simulink model "Velocity_Open_loop"  (R2023a)
settings: Solver=FixedStepAuto  StartTime=0.0  StopTime=10  FixedStep=0.04  RelTol=1e-3
undefined symbols (not defined in the file): Angular, Linear
libraries: robotlib x7
settings Model: Creator=yoav  LastModifiedBy=connectlab
settings OptimizationCC: EnhancedBackFolding=on  PassReuseOutputArgsAs=Individual arguments  ZeroExternalMemoryAtStartup=off  ZeroInternalMemoryAtStartup=off  MaxStackSize=64  OptimizeBlockOrder=speed  DifferentSizesBufferReuse=on  OptimizationCustomize=off  EfficientTunableParamExpr=on
settings DebuggingCC: ParameterTunabilityLossMsg=error
settings HardwareCC: ProdBitPerPointer=32  ProdBitPerSizeT=32  ProdBitPerPtrDiffT=32  ProdLargestAtomicFloat=None  ProdIntDivRoundTo=Undefined  ProdEndianess=Unspecified  ProdWordSize=32  ProdHWDeviceType=Generic->Unspecified (assume 32-bit Generic)
settings SFSimCC: MATLABDynamicMemAlloc=off
settings RTWCC: Description=Embedded Coder  SystemTargetFile=ert.tlc  HardwareBoard=Robot Operating System (ROS)  TLCOptions="-aInlineSetEventsForThisBaseRateFcn=TLC_FALSE -aSuppressMultiTaskScheduler=TLC_FALSE  -aRateBasedStepFcn=0"  TemplateMakefile=ert_default_tmf  Toolchain=Catkin  TargetLang=C++
settings CodeAppCC: ForceParamTrailComments=on  IgnoreCustomStorageClasses=off  OperatorAnnotations=on  SimulinkDataObjDesc=on  SFDataObjDesc=on  InsertBlockDesc=on
settings ERTTargetCC: ExtMode=on  ExtModeMexArgs='192.168.1.155' 0 17725

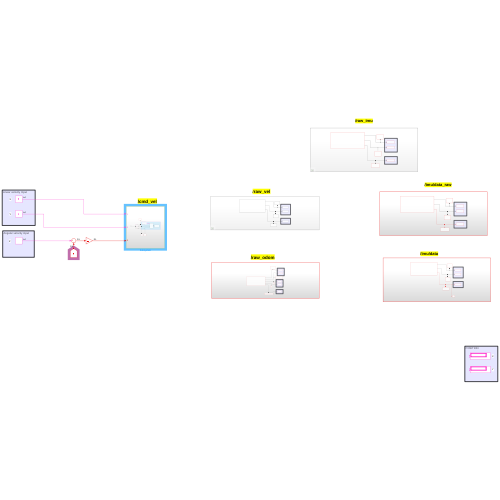
[thumbnail: Simulink's stored preview of the top-level diagram]
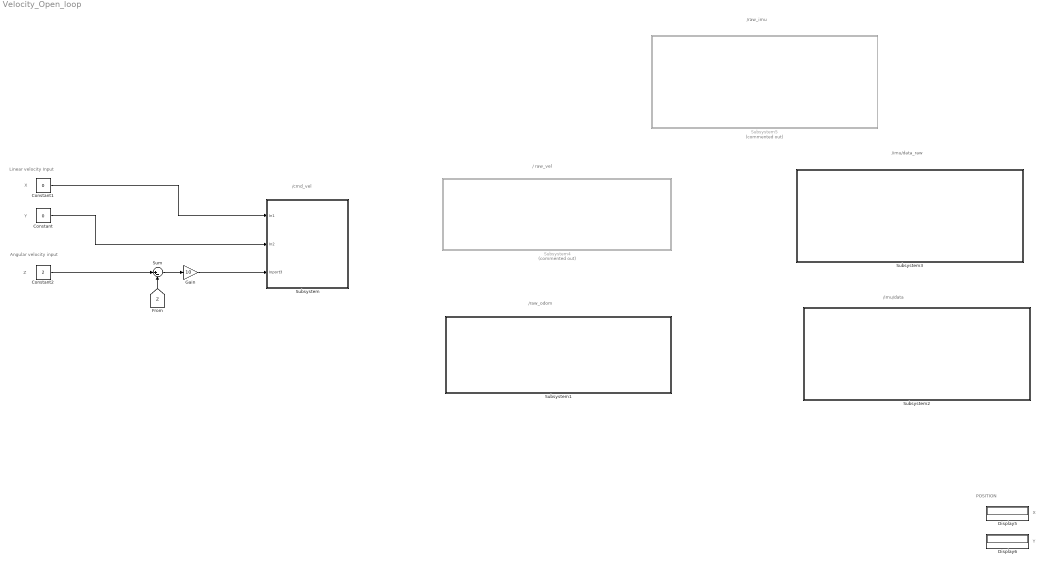
== system Velocity_Open_loop ==
  note: /raw_odom
  note: / raw_vel
  note: X
  note: Y
  note: Z
  note: Linear velocity Input
  note: Angular velocity input
  note: X
  note: POSITION
  note: Y
  note: /cmd_vel
  note: /imu/data_raw
  note: /imu/data
  note: /raw_imu
  Constant : Constant  Value=0
  Constant1 : Constant  Value=0
  Constant2 : Constant  Value=2
  Display5 : Display
  Display6 : Display
  Gain : Gain  Gain=10
  Subsystem : Subsystem
  Subsystem1 : Subsystem
  Subsystem2 : Subsystem
  Subsystem3 : Subsystem
  Subsystem4 : Subsystem  Commented=on
  Subsystem5 : Subsystem  Commented=on
  Sum : Sum  Inputs=|+-
  wires:
  Constant1/1 -> Subsystem/1(In1)
  Constant/1 -> Subsystem/2(In2)
  [Z] -> Sum/2
  Constant2/1 -> Sum/1
  Sum/1 -> Gain/1
  Gain/1 -> Subsystem/3(Inport3)

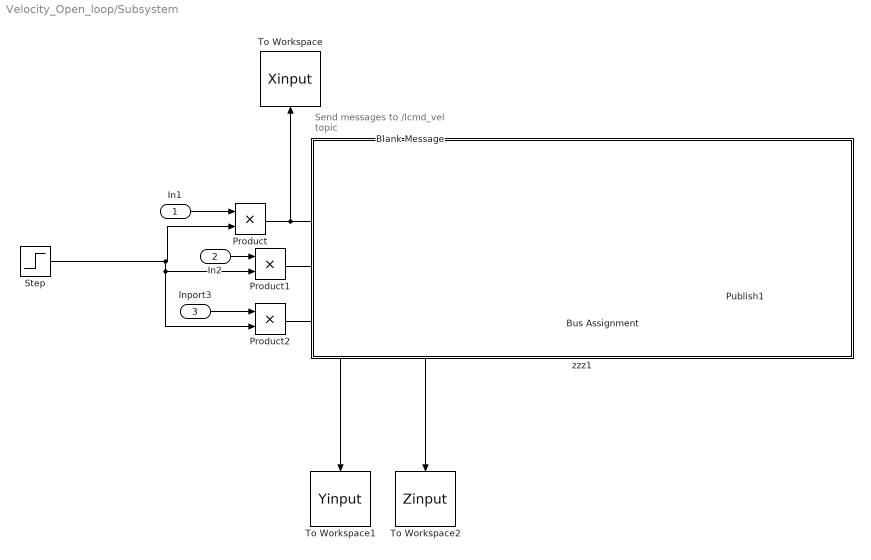
== system Velocity_Open_loop/Subsystem ==
  note: Send messages to /lcmd_vel topic
  In1 : Inport
  In2 : Inport  Port=2
  Inport3 : Inport  Port=3
  Blank Message : robotlib/Blank Message  messageClass=Message  entityType=geometry_msgs/Twist  messageType=geometry_msgs/Twist  SampleTime=inf  legacyBusStruct=off
  Bus Assignment : BusAssignment  AssignedSignals=Linear.X,Linear.Y,Angular.Z
  Product : Product
  Product1 : Product
  Product2 : Product
  Publish1 : robotlib/Publish  topicSource=Specify your own  topic=/cmd_vel  messageType=geometry_msgs/Twist  legacyBusStruct=off  messageQueueLength=105
  Step : Step  SampleTime=0
  To Workspace : ToWorkspace  VariableName=Xinput  SaveFormat=Timeseries  SampleTime=-1
  To Workspace1 : ToWorkspace  VariableName=Yinput  SaveFormat=Timeseries  SampleTime=-1
  To Workspace2 : ToWorkspace  VariableName=Zinput  SaveFormat=Timeseries  SampleTime=-1
  zzz1 : Subsystem  TreatAsAtomicUnit=on
      settings: OpenFcn=% no-op
      mask Display: disp('')
  wires:
  Blank Message/1 -> Bus Assignment/1
  Bus Assignment/1 -> Publish1/1
  In1/1 -> Product/1
  Step/1 -> Product2/2, Product1/2, Product/2
  Product/1 -> Bus Assignment/2, To Workspace/1
  In2/1 -> Product1/1
  Product1/1 -> To Workspace1/1, Bus Assignment/3
  Inport3/1 -> Product2/1
  Product2/1 -> To Workspace2/1, Bus Assignment/4

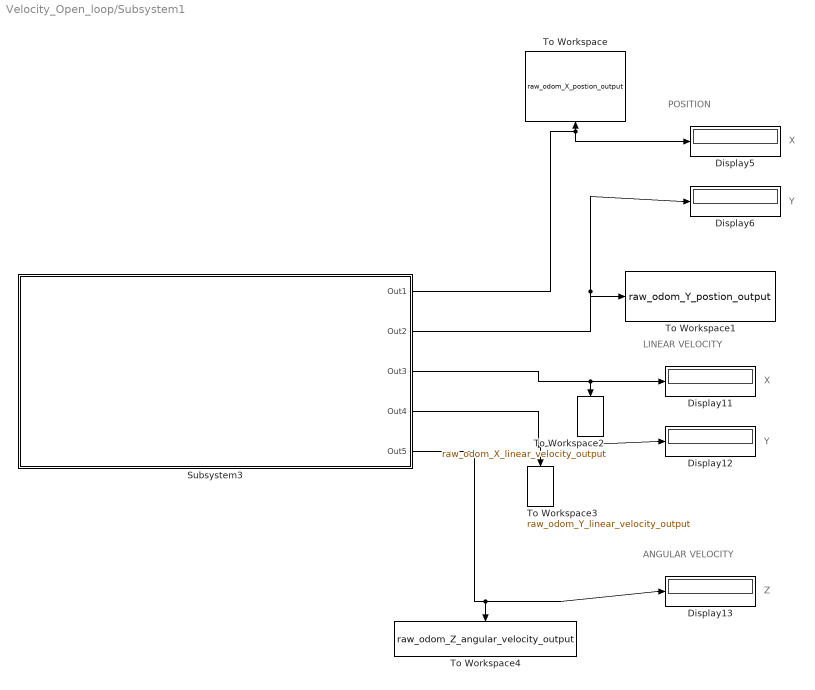
== system Velocity_Open_loop/Subsystem1 ==
  note: LINEAR VELOCITY
  note: X
  note: Y
  note: Z
  note: ANGULAR VELOCITY
  note: X
  note: POSITION
  note: Y
  Display{5..6,11..13} (5 alike) : Display
  Subsystem3 : Subsystem
  To Workspace : ToWorkspace  VariableName=raw_odom_X_postion_output  SaveFormat=Timeseries  SampleTime=-1
  To Workspace1 : ToWorkspace  VariableName=raw_odom_Y_postion_output  SaveFormat=Timeseries  SampleTime=-1
  To Workspace2 : ToWorkspace  VariableName=raw_odom_X_linear_velocity_output  SaveFormat=Timeseries  SampleTime=-1
  To Workspace3 : ToWorkspace  VariableName=raw_odom_Y_linear_velocity_output  SaveFormat=Timeseries  SampleTime=-1
  To Workspace4 : ToWorkspace  VariableName=raw_odom_Z_angular_velocity_output  SaveFormat=Timeseries  SampleTime=-1
  wires:
  Subsystem3/1(Out1) -> Display5/1, To Workspace/1
  Subsystem3/2(Out2) -> Display6/1, To Workspace1/1
  Subsystem3/3(Out3) -> Display11/1, To Workspace2/1
  Subsystem3/4(Out4) -> To Workspace3/1, Display12/1
  Subsystem3/5(Out5) -> Display13/1, To Workspace4/1

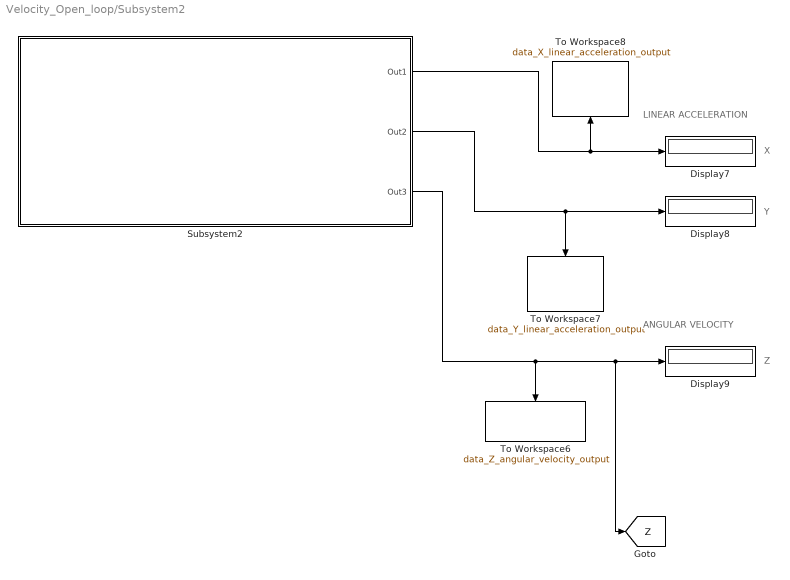
== system Velocity_Open_loop/Subsystem2 ==
  note: Y
  note: Z
  note: LINEAR ACCELERATION
  note: X
  note: ANGULAR VELOCITY
  Display7 : Display
  Display8 : Display
  Display9 : Display
  Subsystem2 : Subsystem
  To Workspace6 : ToWorkspace  VariableName=data_Z_angular_velocity_output  SaveFormat=Timeseries  SampleTime=-1
  To Workspace7 : ToWorkspace  VariableName=data_Y_linear_acceleration_output  SaveFormat=Timeseries  SampleTime=-1
  To Workspace8 : ToWorkspace  VariableName=data_X_linear_acceleration_output  SaveFormat=Timeseries  SampleTime=-1
  tag scope: Z=global
  wires:
  Subsystem2/1(Out1) -> Display7/1, To Workspace8/1
  Subsystem2/2(Out2) -> Display8/1, To Workspace7/1
  Subsystem2/3(Out3) -> To Workspace6/1, [Z], Display9/1

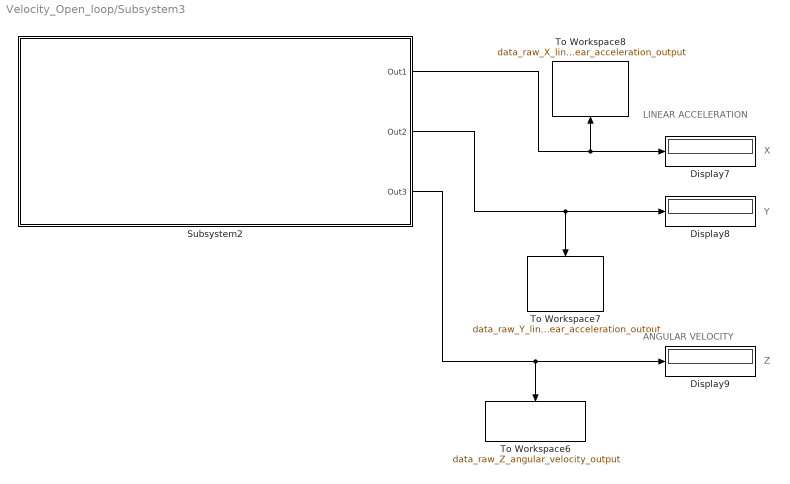
== system Velocity_Open_loop/Subsystem3 ==
  note: Y
  note: Z
  note: LINEAR ACCELERATION
  note: X
  note: ANGULAR VELOCITY
  Display7 : Display
  Display8 : Display
  Display9 : Display
  Subsystem2 : Subsystem
  To Workspace6 : ToWorkspace  VariableName=data_raw_Z_angular_velocity_output  SaveFormat=Timeseries  SampleTime=-1
  To Workspace7 : ToWorkspace  VariableName=data_raw_Y_linear_acceleration_output  SaveFormat=Timeseries  SampleTime=-1
  To Workspace8 : ToWorkspace  VariableName=data_raw_X_linear_acceleration_output  SaveFormat=Timeseries  SampleTime=-1
  wires:
  Subsystem2/1(Out1) -> Display7/1, To Workspace8/1
  Subsystem2/2(Out2) -> Display8/1, To Workspace7/1
  Subsystem2/3(Out3) -> To Workspace6/1, Display9/1

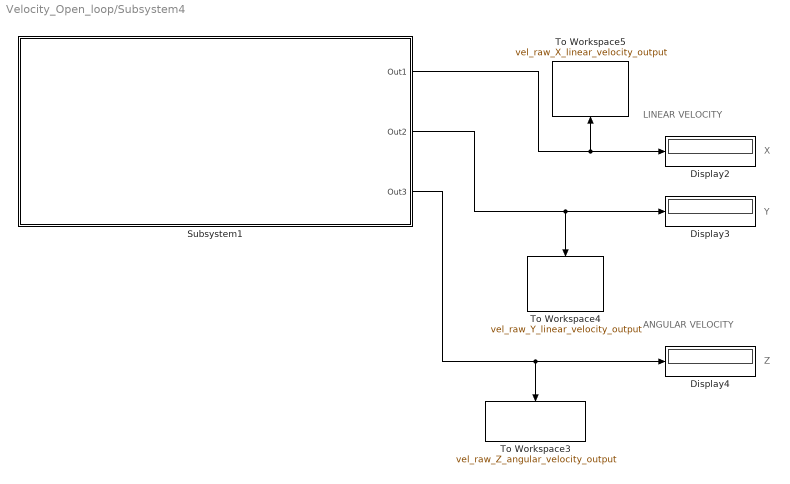
== system Velocity_Open_loop/Subsystem4 ==
  note: LINEAR VELOCITY
  note: X
  note: Y
  note: ANGULAR VELOCITY
  note: Z
  Display2 : Display
  Display3 : Display
  Display4 : Display
  Subsystem1 : Subsystem
  To Workspace3 : ToWorkspace  VariableName=vel_raw_Z_angular_velocity_output  SaveFormat=Timeseries  SampleTime=-1
  To Workspace4 : ToWorkspace  VariableName=vel_raw_Y_linear_velocity_output  SaveFormat=Timeseries  SampleTime=-1
  To Workspace5 : ToWorkspace  VariableName=vel_raw_X_linear_velocity_output  SaveFormat=Timeseries  SampleTime=-1
  wires:
  Subsystem1/2(Out2) -> Display3/1, To Workspace4/1
  Subsystem1/1(Out1) -> Display2/1, To Workspace5/1
  Subsystem1/3(Out3) -> To Workspace3/1, Display4/1

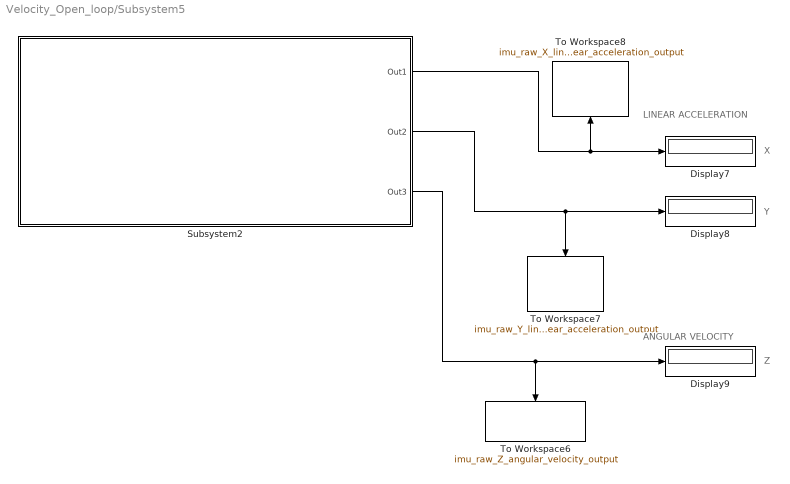
== system Velocity_Open_loop/Subsystem5 ==
  note: Y
  note: Z
  note: LINEAR ACCELERATION
  note: X
  note: ANGULAR VELOCITY
  Display7 : Display
  Display8 : Display
  Display9 : Display
  Subsystem2 : Subsystem
  To Workspace6 : ToWorkspace  VariableName=imu_raw_Z_angular_velocity_output  SaveFormat=Timeseries  SampleTime=-1
  To Workspace7 : ToWorkspace  VariableName=imu_raw_Y_linear_acceleration_output  SaveFormat=Timeseries  SampleTime=-1
  To Workspace8 : ToWorkspace  VariableName=imu_raw_X_linear_acceleration_output  SaveFormat=Timeseries  SampleTime=-1
  wires:
  Subsystem2/1(Out1) -> Display7/1, To Workspace8/1
  Subsystem2/2(Out2) -> Display8/1, To Workspace7/1
  Subsystem2/3(Out3) -> To Workspace6/1, Display9/1

== system Velocity_Open_loop/Subsystem/zzz1 ==

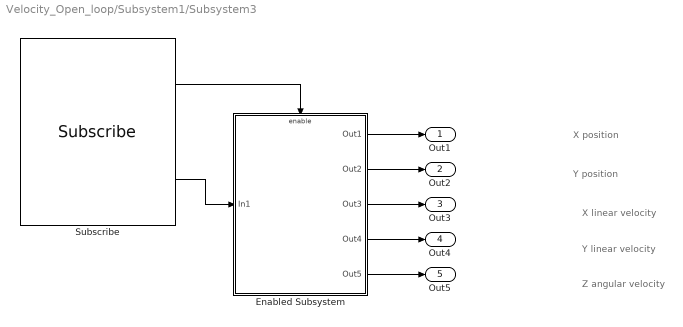
== system Velocity_Open_loop/Subsystem1/Subsystem3 ==
  note: X position
  note: Y position
  note: Z angular velocity
  note: X linear velocity
  note: Y linear velocity
  Enabled Subsystem : Subsystem  TreatAsAtomicUnit=on
  Subscribe : robotlib/Subscribe  topicSource=Select from ROS network  topic=/raw_odom  messageType=nav_msgs/Odometry  SampleTime=-1  legacyBusStruct=off  messageQueueLength=1
      settings: LibrarySourceBlock=roslib/ROS/Subscribe
  Out1 : Outport
  Out2 : Outport  Port=2
  Out3 : Outport  Port=3
  Out4 : Outport  Port=4
  Out5 : Outport  Port=5
  wires:
  Subscribe/2 -> Enabled Subsystem/1(In1)
  Subscribe/1 -> Enabled Subsystem/Enable
  Enabled Subsystem/1(Out1) -> Out1/1
  Enabled Subsystem/2(Out2) -> Out2/1
  Enabled Subsystem/3(Out3) -> Out3/1
  Enabled Subsystem/4(Out4) -> Out4/1
  Enabled Subsystem/5(Out5) -> Out5/1

== system Velocity_Open_loop/Subsystem2/Subsystem2 ==
  note: X linear acceleration
  note: Z angular velocity
  note: Y linear acceleration
  Enabled Subsystem : Subsystem  TreatAsAtomicUnit=on
  Subscribe : robotlib/Subscribe  topicSource=Select from ROS network  topic=/imu/data  messageType=sensor_msgs/Imu  SampleTime=-1  legacyBusStruct=off  messageQueueLength=1
      settings: LibrarySourceBlock=roslib/ROS/Subscribe
  Out1 : Outport
  Out2 : Outport  Port=2
  Out3 : Outport  Port=3
  wires:
  Enabled Subsystem/2(Out8) -> Out2/1
  Subscribe/2 -> Enabled Subsystem/1(In1)
  Enabled Subsystem/1(Out7) -> Out1/1
  Subscribe/1 -> Enabled Subsystem/Enable
  Enabled Subsystem/3(Out9) -> Out3/1

== system Velocity_Open_loop/Subsystem3/Subsystem2 ==
  note: X linear acceleration
  note: Z angular velocity
  note: Y linear acceleration
  Enabled Subsystem : Subsystem  TreatAsAtomicUnit=on
  Subscribe : robotlib/Subscribe  topicSource=Select from ROS network  topic=/imu/data_raw  messageType=sensor_msgs/Imu  SampleTime=-1  legacyBusStruct=off  messageQueueLength=1
      settings: LibrarySourceBlock=roslib/ROS/Subscribe
  Out1 : Outport
  Out2 : Outport  Port=2
  Out3 : Outport  Port=3
  wires:
  Enabled Subsystem/2(Out8) -> Out2/1
  Subscribe/2 -> Enabled Subsystem/1(In1)
  Enabled Subsystem/1(Out7) -> Out1/1
  Subscribe/1 -> Enabled Subsystem/Enable
  Enabled Subsystem/3(Out9) -> Out3/1

== system Velocity_Open_loop/Subsystem4/Subsystem1 ==
  note: X linear velocity
  note: Z angular velocity
  note: Y linear velocity
  Enabled Subsystem : Subsystem  TreatAsAtomicUnit=on
  Subscribe : robotlib/Subscribe  topicSource=Select from ROS network  topic=/raw_vel  messageType=mbs_msgs/Velocities  SampleTime=-1  legacyBusStruct=off  messageQueueLength=1
      settings: LibrarySourceBlock=roslib/ROS/Subscribe
  Out1 : Outport
  Out2 : Outport  Port=2
  Out3 : Outport  Port=3
  wires:
  Enabled Subsystem/2(Out8) -> Out2/1
  Subscribe/2 -> Enabled Subsystem/1(In1)
  Enabled Subsystem/1(Out7) -> Out1/1
  Subscribe/1 -> Enabled Subsystem/Enable
  Enabled Subsystem/3(Out9) -> Out3/1

== system Velocity_Open_loop/Subsystem5/Subsystem2 ==
  note: X linear acceleration
  note: Z angular velocity
  note: Y linear acceleration
  Enabled Subsystem : Subsystem  TreatAsAtomicUnit=on
  Subscribe : robotlib/Subscribe  topicSource=Select from ROS network  topic=/raw_imu  messageType=mbs_msgs/Imu  SampleTime=-1  legacyBusStruct=off  messageQueueLength=1
      settings: LibrarySourceBlock=roslib/ROS/Subscribe
  Out1 : Outport
  Out2 : Outport  Port=2
  Out3 : Outport  Port=3
  wires:
  Enabled Subsystem/2(Out8) -> Out2/1
  Subscribe/2 -> Enabled Subsystem/1(In1)
  Enabled Subsystem/1(Out7) -> Out1/1
  Subscribe/1 -> Enabled Subsystem/Enable
  Enabled Subsystem/3(Out9) -> Out3/1

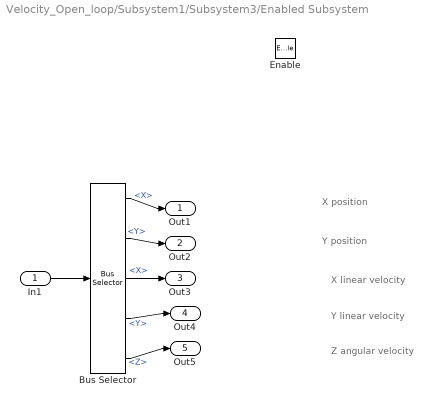
== system Velocity_Open_loop/Subsystem1/Subsystem3/Enabled Subsystem ==
  note: X position
  note: Y position
  note: Z angular velocity
  note: X linear velocity
  note: Y linear velocity
  In1 : Inport
  Enable : EnablePort
  Bus Selector : BusSelector  OutputSignals=Pose.Pose.Position.X,Pose.Pose.Position.Y,Twist.Twist.Linear.X,Twist.Twist.Linear.Y,Twist.Twist.Angular.Z
  Out1 : Outport
  Out2 : Outport  Port=2
  Out3 : Outport  Port=3
  Out4 : Outport  Port=4
  Out5 : Outport  Port=5
  wires:
  In1/1 -> Bus Selector/1
  Bus Selector/1 -> Out1/1  "<X>"
  Bus Selector/2 -> Out2/1  "<Y>"
  Bus Selector/3 -> Out3/1  "<X>"
  Bus Selector/4 -> Out4/1  "<Y>"
  Bus Selector/5 -> Out5/1  "<Z>"

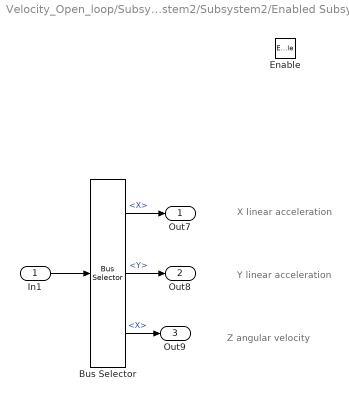
== system Velocity_Open_loop/Subsystem2/Subsystem2/Enabled Subsystem ==
  note: X linear acceleration
  note: Y linear acceleration
  note: Z angular velocity
  In1 : Inport
  Enable : EnablePort
  Bus Selector : BusSelector  OutputSignals=LinearAcceleration.X,LinearAcceleration.Y,AngularVelocity.X
  Out7 : Outport
  Out8 : Outport  Port=2
  Out9 : Outport  Port=3
  wires:
  In1/1 -> Bus Selector/1
  Bus Selector/1 -> Out7/1  "<X>"
  Bus Selector/2 -> Out8/1  "<Y>"
  Bus Selector/3 -> Out9/1  "<X>"

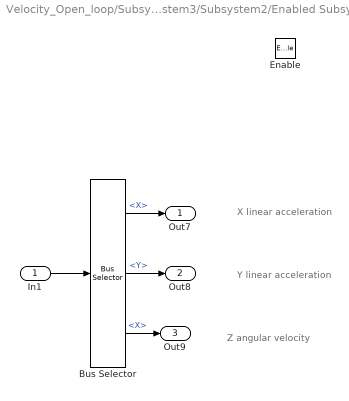
== system Velocity_Open_loop/Subsystem3/Subsystem2/Enabled Subsystem ==
  note: X linear acceleration
  note: Y linear acceleration
  note: Z angular velocity
  In1 : Inport
  Enable : EnablePort
  Bus Selector : BusSelector  OutputSignals=LinearAcceleration.X,LinearAcceleration.Y,AngularVelocity.X
  Out7 : Outport
  Out8 : Outport  Port=2
  Out9 : Outport  Port=3
  wires:
  In1/1 -> Bus Selector/1
  Bus Selector/1 -> Out7/1  "<X>"
  Bus Selector/2 -> Out8/1  "<Y>"
  Bus Selector/3 -> Out9/1  "<X>"

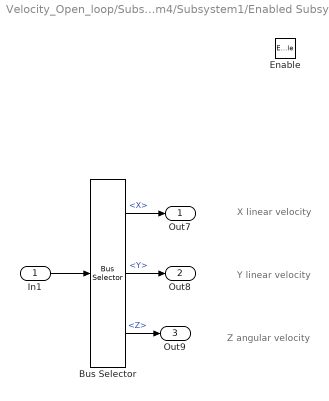
== system Velocity_Open_loop/Subsystem4/Subsystem1/Enabled Subsystem ==
  note: X linear velocity
  note: Y linear velocity
  note: Z angular velocity
  In1 : Inport
  Enable : EnablePort
  Bus Selector : BusSelector  OutputSignals=Linear.X,Linear.Y,Angular.Z
  Out7 : Outport
  Out8 : Outport  Port=2
  Out9 : Outport  Port=3
  wires:
  In1/1 -> Bus Selector/1
  Bus Selector/1 -> Out7/1  "<X>"
  Bus Selector/2 -> Out8/1  "<Y>"
  Bus Selector/3 -> Out9/1  "<Z>"

== system Velocity_Open_loop/Subsystem5/Subsystem2/Enabled Subsystem ==
  note: X linear acceleration
  note: Y linear acceleration
  note: Z angular velocity
  In1 : Inport
  Enable : EnablePort
  Bus Selector : BusSelector  OutputSignals=LinearAcceleration.X,LinearAcceleration.Y,AngularVelocity.Z
  Out7 : Outport
  Out8 : Outport  Port=2
  Out9 : Outport  Port=3
  wires:
  In1/1 -> Bus Selector/1
  Bus Selector/1 -> Out7/1  "<X>"
  Bus Selector/2 -> Out8/1  "<Y>"
  Bus Selector/3 -> Out9/1  "<Z>"
